simulink model "control_model_unstable_jet_1D"  (R2025b)
settings: Solver=VariableStepAuto  StartTime=0.0  StopTime=15000  RelTol=1e-3
values from neighbouring files (symbols this model uses):
  Am = [0 1 0 0; -walpha^2 -2*zeta_alpha*walpha 0 0; 0 0 0 1; 0 0 -wgamma^2 -2*zeta_gamma*wgamma]    [main_v2.m]    (also in script_plane.m = [0 1; -wn^2 -2*zeta*wn])
  B = [0; Cm_delta*K/Iy; 0; 0]    [main_v2.m]    (also in script_plane.m = [0; Cm_delta/Iy])
  Bm = [0; walpha^2; 0; 0]    [main_v2.m]    (also in script_plane.m = [0; wn^2])
  c = 3.2    [main_v2.m]    (also in script_plane.m = 3.45)
  Cm = [1 0 0 0;0 1 0 0; 0 0 0 0; 0 0 0 0]    [main_v2.m]    (also in script_plane.m = [1 0; 0 1])
  Cm_alpha = 0.12    [script_plane.m]
  Cm_alpha_stall = 0.25    [script_plane.m]
  Cm_delta = -0.5    [main_v2.m]    (also in script_plane.m = -1)
  Cm_delta_deep_stall = -0.2    [script_plane.m]
  Cm_delta_stall = -0.5    [script_plane.m]
  Cm_q = -12    [main_v2.m]    (also in script_plane.m = -8)
  delta_max = deg2rad(25)    [main_v2.m]    (also in script_plane.m)
  desired_aoa = deg2rad(45)    [main_v2.m]    (also in script_plane.m = deg2rad(20))
  Dm = zeros(4, 1)    [main_v2.m]    (also in script_plane.m = [0;0])
  gain_e = 0.1    [main_v2.m]    (also in script_plane.m = 50000)
  gain_r = 0.01    [main_v2.m]    (also in script_plane.m = 500000)
  gain_x = 0.00002    (= 2e-05)    [main_v2.m]    (also in script_plane.m = 500000)
  initial_alpha = deg2rad(0)    [main_v2.m]    (also in script_plane.m)
  Iy = 160000    [main_v2.m]    (also in script_plane.m = 70000)
  K = 1/2 *rho * S *c    (= 58.8)    [main_v2.m]    (also in script_plane.m = 1908126.5175)
  Kr = 34.3*10^-3    (= 0.0343)    [main_v2.m]    (also in script_plane.m = -0.825)
  Kx = [19 -8 0 15]*10^-5    [main_v2.m]    (also in script_plane.m = [1.33 0.15])
  P = lyap(Am',Q)    [main_v2.m]    (also in script_plane.m)
  sigma_r = 0.001    [main_v2.m]    (also in script_plane.m = 0.0002)
  sigma_w = 0.001    [main_v2.m]    (also in script_plane.m = 0.0002)
  sigma_x = 0.001    [main_v2.m]    (also in script_plane.m = 0.0002)
  speed = 180    [main_v2.m]    (also in script_plane.m)
libraries: simulink_extras x11, slctrl_adaptive x1
settings Model: Creator=marti  LastModifiedBy=marti

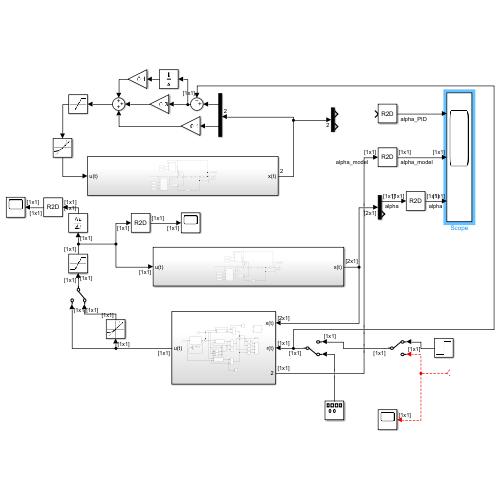
[thumbnail: Simulink's stored preview of the top-level diagram]
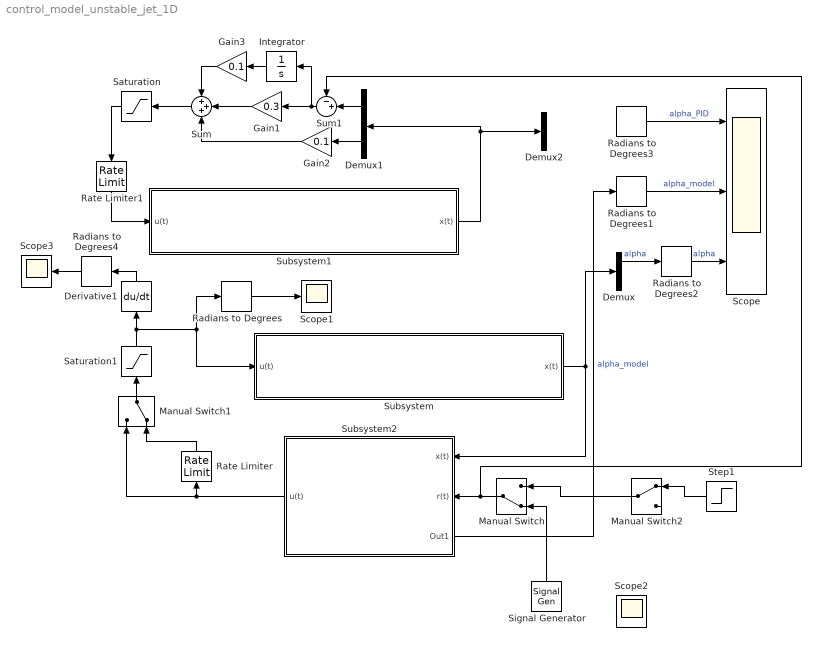
== system control_model_unstable_jet_1D ==
  Demux : Demux  Outputs=2
  Demux1 : Demux  Outputs=2
  Demux2 : Demux  Outputs=2
  Derivative1 : Derivative
  Gain1 : Gain  Gain=0.3
  Gain2 : Gain  Gain=0.1
  Gain3 : Gain  Gain=0.1
  Integrator : Integrator
  Manual Switch : ManualSwitch  CurrentSetting=0
  Manual Switch1 : ManualSwitch  CurrentSetting=0
  Manual Switch2 : ManualSwitch
  Radians to Degrees{,1..4} (5 alike) : simulink_extras/Transformations/Radians to Degrees
  Rate Limiter : RateLimiter  RisingSlewLimit=deg2rad(40)  FallingSlewLimit=-deg2rad(40)  SampleTimeMode=inherited
  Rate Limiter1 : RateLimiter  RisingSlewLimit=deg2rad(60)  FallingSlewLimit=-deg2rad(60)  SampleTimeMode=inherited
  Saturation : Saturate  UpperLimit=delta_max  LowerLimit=-delta_max
  Saturation1 : Saturate  UpperLimit=delta_max  LowerLimit=-delta_max
  Scope : Scope  NumInputPorts=3
      settings: ActiveDisplayYMinimum=-25.162431052261546  ActiveDisplayYMaximum=25.164915879658963  DataLoggingVariableName=ScopeData3
  Scope1 : Scope
      settings: ActiveDisplayYMinimum=-11.955664071960936  ActiveDisplayYMaximum=11.734788534525411  DataLoggingVariableName=ScopeData5
  Scope2 : Scope
      settings: ActiveDisplayYMinimum=-1.2499999999415519  ActiveDisplayYMaximum=1.2499999999935056  DataLoggingVariableName=ScopeData10
  Scope3 : Scope
      settings: ActiveDisplayYMinimum=-75.000000000000327  ActiveDisplayYMaximum=75.000000000000327  DataLoggingVariableName=ScopeData11
  Signal Generator : SignalGenerator  WaveForm=square  Amplitude=desired_aoa  Frequency=0.5  Units=rad/sec
  Step1 : Step  After=desired_aoa  SampleTime=0
  Subsystem : Subsystem
  Subsystem1 : Subsystem
  Subsystem2 : Subsystem
      settings: PortSchema="{\"entries\":[{\"content\":{\"sides\":[{\"content\":{\"connectorIds\":[\"Out2\",\"In1\",\"In2\"]},\"type\":\"ConnectorPlacement.EquallySpacedRectSide\",\"uuid\":\"2a5405b8-f474-466f-9064-f86b75893dd0\"},{\"content\":{\"connectorIds\":[\"Out1\"],\"side\":\"RIGHT\"},\"type\":\"ConnectorPlacement.EquallySpacedRectSide\",\"uuid\":\"ad673661-f4e9-494b-83cc-7452eec3fe31\"},{\"content\":{\"side\":\"TOP\"},\"type\":\"ConnectorPlacement.EquallySpacedRectSide\",\"uuid\":\"21a76317-3288-4ff3-bd02-68708e86e3a8\"}]},\"type\":\"ConnectorPlacement.EquallySpacedConnector\",\"uuid\":\"fc0ce599-928f-4c66-9629-0b98f2391e21\"}],\"packageUris\":[\"http://schema.mathworks.com/mf0/Connector/R2020b\"],\"version\":\"1.0\"}"
  Sum : Sum  Inputs=+++
  Sum1 : Sum  Inputs=-+|
  wires:
  Signal Generator/1 -> Manual Switch/2
  Radians to Degrees/1 -> Scope1/1
  Sum/1 -> Saturation/1
  Saturation/1 -> Rate Limiter1/1
  Subsystem2/2(Out1) -> Radians to Degrees1/1  "alpha_model"
  Demux/1 -> Radians to Degrees2/1  "alpha"
  Demux1/2 -> Gain2/1
  Sum1/1 -> Integrator/1, Gain1/1
  Demux1/1 -> Sum1/2
  Subsystem/1(x(t)) -> Subsystem2/2(x(t)), Demux/1
  Manual Switch/1 -> Sum1/1, Subsystem2/1(r(t))
  Rate Limiter1/1 -> Subsystem1/1(u(t))
  Subsystem1/1(x(t)) -> Demux1/1, Demux2/1
  Radians to Degrees2/1 -> Scope/3  "alpha"
  Radians to Degrees1/1 -> Scope/2  "alpha_model"
  Radians to Degrees3/1 -> Scope/1  "alpha_PID"
  Saturation1/1 -> Subsystem/1(u(t)), Radians to Degrees/1, Derivative1/1
  Subsystem2/1(u(t)) -> Manual Switch1/1, Rate Limiter/1
  Manual Switch1/1 -> Saturation1/1
  Rate Limiter/1 -> Manual Switch1/2
  Gain1/1 -> Sum/2
  Gain2/1 -> Sum/3
  Integrator/1 -> Gain3/1
  Gain3/1 -> Sum/1
  Manual Switch2/1 -> Manual Switch/1
  Step1/1 -> Manual Switch2/1
  ? -> Scope2/1, Manual Switch2/2
  Derivative1/1 -> Radians to Degrees4/1
  Radians to Degrees4/1 -> Scope3/1

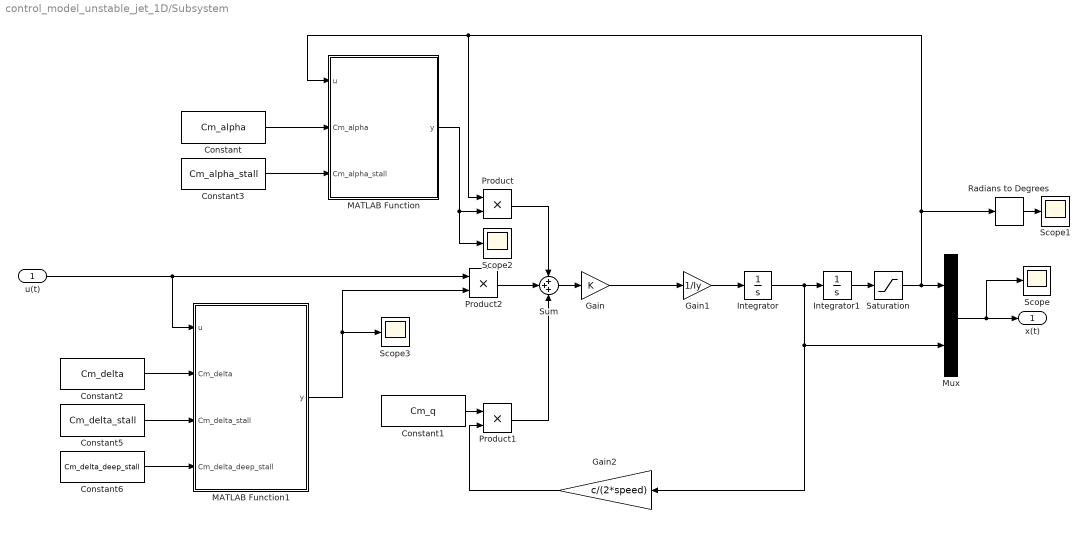
== system control_model_unstable_jet_1D/Subsystem ==
  u(t) : Inport
  Constant : Constant  Value=Cm_alpha
  Constant1 : Constant  Value=Cm_q
  Constant2 : Constant  Value=Cm_delta
  Constant3 : Constant  Value=Cm_alpha_stall
  Constant5 : Constant  Value=Cm_delta_stall
  Constant6 : Constant  Value=Cm_delta_deep_stall
  Gain : Gain  Gain=K
  Gain1 : Gain  Gain=1/Iy
  Gain2 : Gain  Gain=c/(2*speed)
  Integrator : Integrator
  Integrator1 : Integrator  InitialCondition=initial_alpha
  MATLAB Function : MATLAB Function  TreatAsAtomicUnit=on
  MATLAB Function1 : MATLAB Function  TreatAsAtomicUnit=on
  Mux : Mux  Inputs=2
  Product : Product
  Product1 : Product
  Product2 : Product
  Radians to Degrees : simulink_extras/Transformations/Radians to Degrees
  Saturation : Saturate  UpperLimit=deg2rad(80)  LowerLimit=-deg2rad(80)
  Scope{,1..3} (4 alike) : Scope
      Scope1 settings: ActiveDisplayYMinimum=-1  ActiveDisplayYMaximum=1
      Scope2 settings: ActiveDisplayYMinimum=0.10375000000000001  ActiveDisplayYMaximum=0.26625  DataLoggingVariableName=ScopeData2
      Scope3 settings: ActiveDisplayYMinimum=-1  ActiveDisplayYMaximum=1  DataLoggingVariableName=ScopeData4
  Sum : Sum  Inputs=+++
  x(t) : Outport
  wires:
  Constant/1 -> MATLAB Function/2(Cm_alpha)
  Gain/1 -> Gain1/1
  Radians to Degrees/1 -> Scope1/1
  Mux/1 -> x(t)/1, Scope/1
  Product2/1 -> Sum/2
  Sum/1 -> Gain/1
  Gain1/1 -> Integrator/1
  Integrator/1 -> Gain2/1, Mux/2, Integrator1/1
  Constant1/1 -> Product1/1
  Product1/1 -> Sum/3
  MATLAB Function/1(y) -> Scope2/1, Product/2
  Product/1 -> Sum/1
  Constant6/1 -> MATLAB Function1/4(Cm_delta_deep_stall)
  u(t)/1 -> Product2/1, MATLAB Function1/1(u)
  Gain2/1 -> Product1/2
  Constant3/1 -> MATLAB Function/3(Cm_alpha_stall)
  Constant2/1 -> MATLAB Function1/2(Cm_delta)
  MATLAB Function1/1(y) -> Product2/2, Scope3/1
  Constant5/1 -> MATLAB Function1/3(Cm_delta_stall)
  Integrator1/1 -> Saturation/1
  Saturation/1 -> Product/1, MATLAB Function/1(u), Radians to Degrees/1, Mux/1

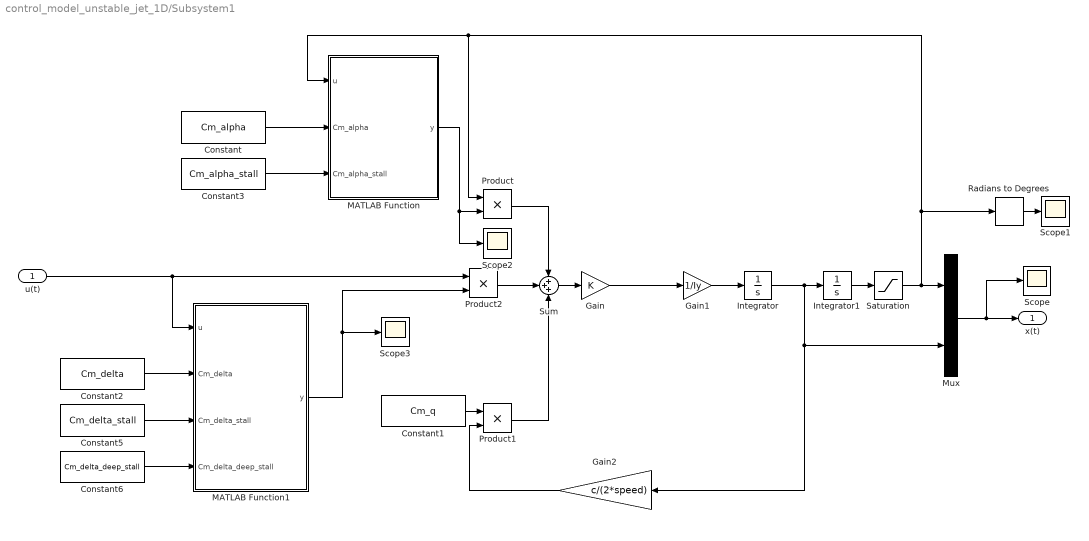
== system control_model_unstable_jet_1D/Subsystem1 ==
  u(t) : Inport
  Constant : Constant  Value=Cm_alpha
  Constant1 : Constant  Value=Cm_q
  Constant2 : Constant  Value=Cm_delta
  Constant3 : Constant  Value=Cm_alpha_stall
  Constant5 : Constant  Value=Cm_delta_stall
  Constant6 : Constant  Value=Cm_delta_deep_stall
  Gain : Gain  Gain=K
  Gain1 : Gain  Gain=1/Iy
  Gain2 : Gain  Gain=c/(2*speed)
  Integrator : Integrator
  Integrator1 : Integrator  InitialCondition=initial_alpha
  MATLAB Function : MATLAB Function  TreatAsAtomicUnit=on
  MATLAB Function1 : MATLAB Function  TreatAsAtomicUnit=on
  Mux : Mux  Inputs=2
  Product : Product
  Product1 : Product
  Product2 : Product
  Radians to Degrees : simulink_extras/Transformations/Radians to Degrees
  Saturation : Saturate  UpperLimit=deg2rad(80)  LowerLimit=-deg2rad(80)
  Scope{,1..3} (4 alike) : Scope
      Scope1 settings: ActiveDisplayYMinimum=-1  ActiveDisplayYMaximum=1
      Scope2 settings: ActiveDisplayYMinimum=-1  ActiveDisplayYMaximum=1  DataLoggingVariableName=ScopeData2
      Scope3 settings: ActiveDisplayYMinimum=-1  ActiveDisplayYMaximum=1  DataLoggingVariableName=ScopeData4
  Sum : Sum  Inputs=+++
  x(t) : Outport
  wires:
  Constant/1 -> MATLAB Function/2(Cm_alpha)
  Gain/1 -> Gain1/1
  Radians to Degrees/1 -> Scope1/1
  Mux/1 -> x(t)/1, Scope/1
  Product2/1 -> Sum/2
  Sum/1 -> Gain/1
  Gain1/1 -> Integrator/1
  Integrator/1 -> Gain2/1, Mux/2, Integrator1/1
  Constant1/1 -> Product1/1
  Product1/1 -> Sum/3
  MATLAB Function/1(y) -> Scope2/1, Product/2
  Product/1 -> Sum/1
  Constant6/1 -> MATLAB Function1/4(Cm_delta_deep_stall)
  u(t)/1 -> Product2/1, MATLAB Function1/1(u)
  Gain2/1 -> Product1/2
  Constant3/1 -> MATLAB Function/3(Cm_alpha_stall)
  Constant2/1 -> MATLAB Function1/2(Cm_delta)
  MATLAB Function1/1(y) -> Product2/2, Scope3/1
  Constant5/1 -> MATLAB Function1/3(Cm_delta_stall)
  Integrator1/1 -> Saturation/1
  Saturation/1 -> Product/1, MATLAB Function/1(u), Radians to Degrees/1, Mux/1

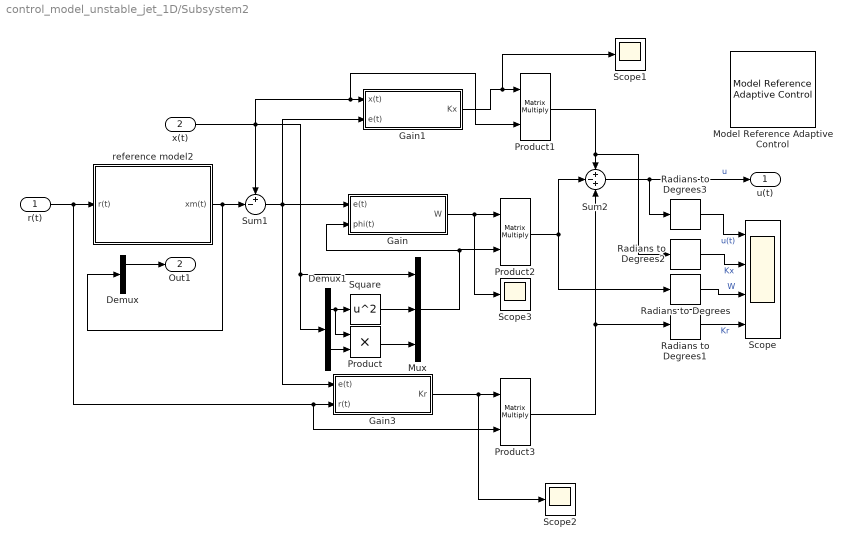
== system control_model_unstable_jet_1D/Subsystem2 ==
  r(t) : Inport
  x(t) : Inport  Port=2  PortDimensions=[2 1]
  Demux : Demux  Outputs=2
  Demux1 : Demux  Outputs=2
  Gain : Subsystem
  Gain1 : Subsystem
  Gain3 : Subsystem
  Model Reference Adaptive Control : slctrl_adaptive/Model Reference Adaptive Control  selectType=Direct  A=0  B=1  Ahat=0  ALrEnable=on  gamma_a=1  ALrEnableMod=on  Bhat=1  BLrEnable=on  gamma_b=1  BLrEnableMod=on  externalKtauEnable=off  k_tau=-1  estParamOutput=off  Am=-1  Bm=1  kx=0  FBLrEnable=on  gamma_kx=1  FBLrEnableMod=on  kr=0  FFLrEnable=on  gamma_kr=1  FFLrEnableMod=on  AdaptEnable=on  gamma=1  WLrEnableMod=on  Q=1  FeatureTypeOptions=State  shlHiddenLayerSize=10  gamma_V=0.1  nCen=20  cSpanMin=-1  cSpanMax=1  cSig=5  adaptiveCntrlOutport=off  modChoice=None  sigma_val=0.1  DiscreteEnable=off  Ts=0.05  IntegrationMethods=Forward Euler
      settings: LibrarySourceBlock=slctrlblks/Adaptive Control/Model Reference Adaptive Control
  Mux : Mux  Inputs=3
  Product : Product
  Product1 : Product  Multiplication=Matrix(*)
  Product2 : Product  Multiplication=Matrix(*)
  Product3 : Product  Multiplication=Matrix(*)
  Radians to Degrees{,1..3} (4 alike) : simulink_extras/Transformations/Radians to Degrees
  Scope : Scope  NumInputPorts=4
      settings: ActiveDisplayYMinimum=-9.0682862927910186  ActiveDisplayYMaximum=9.0335526563219037  DataLoggingVariableName=ScopeData6
  Scope1 : Scope
      settings: ActiveDisplayYMinimum=0.0047092612949780274  ActiveDisplayYMaximum=0.45412293934895304  DataLoggingVariableName=ScopeData7
  Scope2 : Scope
      settings: ActiveDisplayYMinimum=-0.17021830796755916  ActiveDisplayYMaximum=-0.018035228291967735  DataLoggingVariableName=ScopeData8
  Scope3 : Scope
      settings: ActiveDisplayYMinimum=-0.004053735847054353  ActiveDisplayYMaximum=0.00070829013075868132  DataLoggingVariableName=ScopeData9
  Square : Math  Operator=square
  Sum1 : Sum  Inputs=+-|
  Sum2 : Sum  Inputs=+-+
  reference model2 : Subsystem  TreatAsAtomicUnit=on
  u(t) : Outport
  Out1 : Outport  Port=2
  wires:
  r(t)/1 -> Product3/2, Gain3/2(r(t)), reference model2/1(r(t))
  reference model2/1(xm(t)) -> Sum1/2, Demux/1
  x(t)/1 -> Demux1/1, Mux/1, Product1/2, Gain1/1(x(t)), Sum1/1
  Sum1/1 -> Gain/1(e(t)), Gain1/2(e(t)), Gain3/1(e(t))
  Product1/1 -> Radians to Degrees2/1, Sum2/1
  Gain/1(W) -> Scope3/1, Product2/1
  Demux/1 -> Out1/1
  Gain1/1(Kx) -> Scope1/1, Product1/1
  Gain3/1(Kr) -> Scope2/1, Product3/1
  Product3/1 -> Sum2/3, Radians to Degrees1/1
  Demux1/1 -> Product/1, Square/1
  Square/1 -> Mux/2
  Product/1 -> Mux/3
  Demux1/2 -> Product/2
  Mux/1 -> Product2/2, Gain/2(phi(t))
  Product2/1 -> Radians to Degrees/1, Sum2/2
  Radians to Degrees2/1 -> Scope/2  "Kx"
  Radians to Degrees/1 -> Scope/3  "W"
  Radians to Degrees1/1 -> Scope/4  "Kr"
  Sum2/1 -> Radians to Degrees3/1, u(t)/1  "u"
  Radians to Degrees3/1 -> Scope/1  "u(t)"

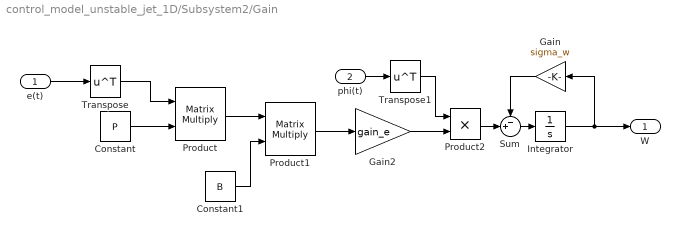
== system control_model_unstable_jet_1D/Subsystem2/Gain ==
  e(t) : Inport
  phi(t) : Inport  Port=2
  Constant : Constant  Value=P  VectorParams1D=off
  Constant1 : Constant  Value=B  VectorParams1D=off
  Gain : Gain  Gain=sigma_w
  Gain2 : Gain  Gain=gain_e
  Integrator : Integrator
  Product : Product  Multiplication=Matrix(*)
  Product1 : Product  Multiplication=Matrix(*)
  Product2 : Product
  Sum : Sum  Inputs=-+|
  Transpose : Math  Operator=transpose
  Transpose1 : Math  Operator=transpose
  W : Outport
  wires:
  Product1/1 -> Gain2/1
  Product/1 -> Product1/1
  Constant1/1 -> Product1/2
  Gain2/1 -> Product2/2
  e(t)/1 -> Transpose/1
  Constant/1 -> Product/2
  Transpose/1 -> Product/1
  Integrator/1 -> Gain/1, W/1
  phi(t)/1 -> Transpose1/1
  Transpose1/1 -> Product2/1
  Product2/1 -> Sum/2
  Sum/1 -> Integrator/1
  Gain/1 -> Sum/1

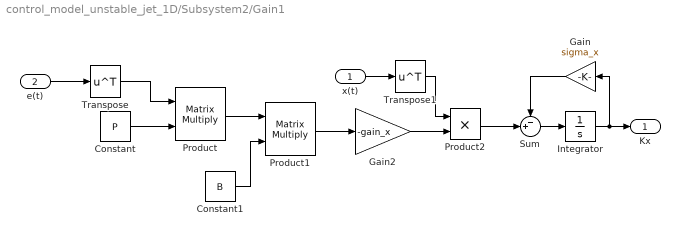
== system control_model_unstable_jet_1D/Subsystem2/Gain1 ==
  x(t) : Inport
  e(t) : Inport  Port=2
  Constant : Constant  Value=P  VectorParams1D=off
  Constant1 : Constant  Value=B  VectorParams1D=off
  Gain : Gain  Gain=sigma_x
  Gain2 : Gain  Gain=-gain_x
  Integrator : Integrator  InitialCondition=Kx
  Product : Product  Multiplication=Matrix(*)
  Product1 : Product  Multiplication=Matrix(*)
  Product2 : Product
  Sum : Sum  Inputs=-+|
  Transpose : Math  Operator=transpose
  Transpose1 : Math  Operator=transpose
  Kx : Outport
  wires:
  Product1/1 -> Gain2/1
  Product/1 -> Product1/1
  Constant1/1 -> Product1/2
  Gain2/1 -> Product2/2
  e(t)/1 -> Transpose/1
  Constant/1 -> Product/2
  Transpose/1 -> Product/1
  Integrator/1 -> Gain/1, Kx/1
  x(t)/1 -> Transpose1/1
  Transpose1/1 -> Product2/1
  Sum/1 -> Integrator/1
  Product2/1 -> Sum/2
  Gain/1 -> Sum/1

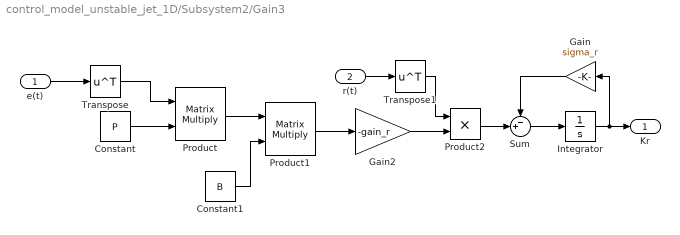
== system control_model_unstable_jet_1D/Subsystem2/Gain3 ==
  e(t) : Inport
  r(t) : Inport  Port=2
  Constant : Constant  Value=P  VectorParams1D=off
  Constant1 : Constant  Value=B  VectorParams1D=off
  Gain : Gain  Gain=sigma_r
  Gain2 : Gain  Gain=-gain_r
  Integrator : Integrator  InitialCondition=Kr
  Product : Product  Multiplication=Matrix(*)
  Product1 : Product  Multiplication=Matrix(*)
  Product2 : Product
  Sum : Sum  Inputs=-+|
  Transpose : Math  Operator=transpose
  Transpose1 : Math  Operator=transpose
  Kr : Outport
  wires:
  Product1/1 -> Gain2/1
  Product/1 -> Product1/1
  Constant1/1 -> Product1/2
  Gain2/1 -> Product2/2
  e(t)/1 -> Transpose/1
  Constant/1 -> Product/2
  Transpose/1 -> Product/1
  Integrator/1 -> Gain/1, Kr/1
  r(t)/1 -> Transpose1/1
  Transpose1/1 -> Product2/1
  Sum/1 -> Integrator/1
  Product2/1 -> Sum/2
  Gain/1 -> Sum/1

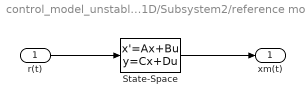
== system control_model_unstable_jet_1D/Subsystem2/reference model2 ==
  r(t) : Inport
  State-Space : StateSpace  A=Am  B=Bm  C=Cm  D=Dm  InitialCondition=[0;0]
  xm(t) : Outport  PortDimensions=[2 1]
  wires:
  State-Space/1 -> xm(t)/1
  r(t)/1 -> State-Space/1

== matlab function control_model_unstable_jet_1D/Subsystem/MATLAB Function1 ==
  data: u input; y output; Cm_delta input; Cm_delta_stall input; Cm_delta_deep_stall input
function y = fcn(u, Cm_delta, Cm_delta_stall, Cm_delta_deep_stall)
if abs(u)<deg2rad(12)
    y=Cm_delta;
elseif abs(u)<deg2rad(20)
    y=Cm_delta_stall;
else
    y=Cm_delta_deep_stall;
end

== matlab function control_model_unstable_jet_1D/Subsystem/MATLAB Function ==
  data: u input; y output; Cm_alpha input; Cm_alpha_stall input
function y = fcn(u, Cm_alpha, Cm_alpha_stall)
if abs(u)<deg2rad(15)
    y=Cm_alpha;
else
    y=Cm_alpha_stall;
end

== matlab function control_model_unstable_jet_1D/Subsystem1/MATLAB Function ==
  data: u input; y output; Cm_alpha input; Cm_alpha_stall input
function y = fcn(u, Cm_alpha, Cm_alpha_stall)
if abs(u)<deg2rad(15)
    y=Cm_alpha;
else
    y=Cm_alpha_stall;
end

== matlab function control_model_unstable_jet_1D/Subsystem1/MATLAB Function1 ==
  data: u input; y output; Cm_delta input; Cm_delta_stall input; Cm_delta_deep_stall input
function y = fcn(u, Cm_delta, Cm_delta_stall, Cm_delta_deep_stall)
if abs(u)<deg2rad(12)
    y=Cm_delta;
elseif abs(u)<deg2rad(20)
    y=Cm_delta_stall;
else
    y=Cm_delta_deep_stall;
end
